simulink model "scdmechconveyor"  (Simulink 7.6)
settings: Solver=ode45  StartTime=0  StopTime=20  FixedStep=0.1  RelTol=1e-4  AbsTol=1e-6
model workspace (MAT data in the model file):
  Dk = [0 0 -1]
  Ck = [-0.0984238285661 -0.00713806743411 0.066683215581 0.191712430065 -0.740222532454]
  Bk = [-1142.96829869  0  0; -16827.8569202  22530.9100751  0; -891.017707814  1697.05627485  0; -295.52924747  169.705627485  0; -37.2617766448  6.32455532034  0]
  Ak = [-108.803869467  1  0  0  0; -1589.64026344  0  -597.440973765  -5974.40973765  17812.2483984; -84.8196529029  0  -50  -450  1341.6407865; -28.1326487378  0  0  -50  134.16407865; -3.54710230093  0  0  0  0]
  Dw = 800
  Cw = [-21.2132034356 -212.132034356 632.455532034]
  Bw = [1697.05627485; 169.705627485; 6.32455532034]
  Aw = [-50  -450  1341.6407865; 0  -50  134.16407865; 0  0  0]
  Dwinv = 0.00125
  Cwinv = [-0.0265165042945 -0.265165042945 0.790569415042]
  Bwinv = [-2.12132034356; -0.212132034356; -0.00790569415042]
  Awinv = [-5  0  0; 4.5  -5  0; 0.167705098312  1.67705098312  -5]
  Sig : Simulink.Signal (value not decoded)
values from neighbouring files (symbols this model uses):
  m = 0.1    [magballdat.m]
libraries: mblibv1 x18
settings Model: Creator=The MathWorks Inc.  ExtModeAutoUpdateStatusClock=off
settings SolverCC: InsertRTBMode=Auto
settings DataIOCC: SaveOutput=off  SaveTime=off  SignalLoggingName=scd_datalog
settings OptimizationCC: BooleanDataType=off  InlineInvariantSignals=on  InitFltsAndDblsToZero=on
settings DebuggingCC: AlgebraicLoopMsg=none  SaveWithParameterizedLinksMsg=none  CheckExecutionContextPreStartOutputMsg=on  CheckExecutionContextRuntimeOutputMsg=on  SignalResolutionControl=TryResolveAllWithWarning  SolverPrmCheckMsg=none  MultiTaskDSMMsg=warning  UnconnectedInputMsg=none  UnconnectedOutputMsg=none  UnconnectedLineMsg=none  InitInArrayFormatMsg=none  StrictBusMsg=None
settings HardwareCC: TargetUnknown=on
settings GRTTargetCC: TargetFcnLib=ansi_tfl_tmw.mat
settings SimMechanicsCC: WarnOnRedundantConstraints=off

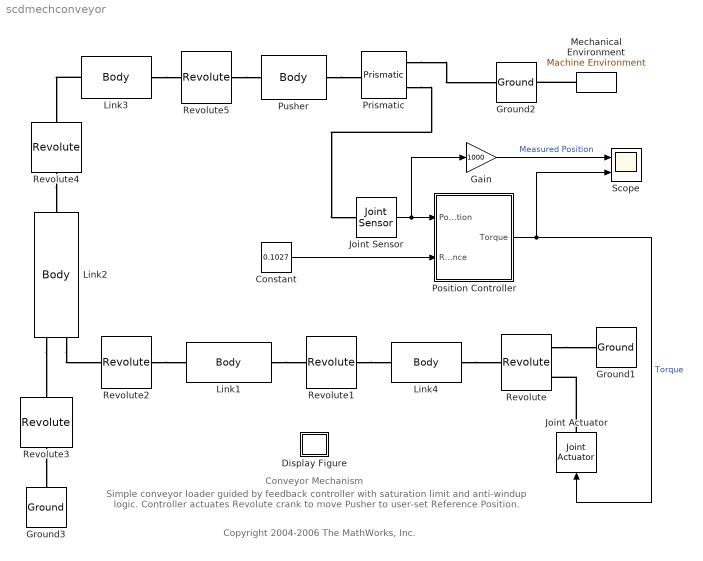
== system scdmechconveyor ==
  note: Conveyor Mechanism
  note: Simple conveyor loader guided by feedback controller with saturation limit
      | and anti-windup logic. Controller actuates Revolute crank to move Pusher
      | to user-set Reference Position.
  note: Copyright 2004-2006 The MathWorks, Inc.
  Constant : Constant  Value=0.1027
  Display Figure : Subsystem  Tag=Help  Description="Help callback for conveyor model: mech_conveyor.  Opens Help browser to Type 19 marker at documentation for this tutorial model."
      settings: OpenFcn=pmhelpview([docroot '/toolbox/physmod/mech/mech.map'], 'mech_conveyor_help');
      mask Type: Help callback
      mask Display: image(imread('info.bmp'))
  Gain : Gain  Gain=1000  SaturateOnIntegerOverflow=on  OutDataTypeStr=Inherit: Same as input  ParamDataTypeStr=Inherit: Same as input
  Ground1 : mblibv1/Bodies/Ground  DialogController=MECH.DynMechDlgSource  SystemSampleTime=-1  UpdateFromCAD=off  LeftPortType=env  RightPortType=workingframe  PhysicalDomain=Mechanical  DialogClass=GroundBlock  CoordPosition=[0.280 0.210 0]  CoordPositionUnits=m  StateVectorMgrId=-1  MachineId=[0 0]  ShowEnvPort=off
  Ground2 : mblibv1/Bodies/Ground  DialogController=MECH.DynMechDlgSource  SystemSampleTime=-1  UpdateFromCAD=off  LeftPortType=env  RightPortType=workingframe  PhysicalDomain=Mechanical  DialogClass=GroundBlock  CoordPosition=[0.412 0.5 0]  CoordPositionUnits=m  StateVectorMgrId=-1  MachineId=[0 0]  ShowEnvPort=on
  Ground3 : mblibv1/Bodies/Ground  DialogController=MECH.DynMechDlgSource  SystemSampleTime=-1  UpdateFromCAD=off  LeftPortType=env  RightPortType=workingframe  PhysicalDomain=Mechanical  DialogClass=GroundBlock  CoordPosition=[0.08 0.11 0]  CoordPositionUnits=m  StateVectorMgrId=-1  MachineId=[0 0]  ShowEnvPort=off
  Joint Actuator : mblibv1/Sensors &  Actuators/Joint Actuator  DialogController=MECH.DynMechDlgSource  SystemSampleTime=-1  UpdateFromCAD=off  PhysicalDomain=Mechanical  PortType=blob  ActuationStyle=Force  AngleUnits=rad  ArcVelocityUnits=rad/s  ArcAccelerationUnits=rad/s^2  CoordPositionUnits=m  VelocityUnits=m/s  AccelerationUnits=m/s^2  ForceUnits=N  TorqueUnits=N-m  ActiveIO=on  Width=1  DialogClass=MechanicalActuatorBlock  Primitive=R1  ReferenceFrame=Absolute (INERTIAL)
  Joint Sensor : mblibv1/Sensors &  Actuators/Joint Sensor  DialogController=MECH.DynMechDlgSource  SystemSampleTime=-1  UpdateFromCAD=off  PhysicalDomain=Mechanical  PortType=blob  Muxed=on  Pose=off  Angle=on  AngleUnits=deg  ArcVelocity=off  ArcVelocityUnits=deg/s  ArcAcceleration=off  ArcAccelerationUnits=deg/s^2  CoordPosition=on  CoordPositionUnits=m  Velocity=off  VelocityUnits=m/s  Acceleration=off  AccelerationUnits=m/s^2  Quaternion=on  QuaternionDT=off  QuaternionDDT=off  QuaternionUnits=off  OutputVector=[ 1 ]  ActiveIO=on  Width=1  DialogClass=MechanicalSensorBlock  Primitive=P1  Force=off  ForceUnits=N  Torque=off  TorqueUnits=N-m  ReferenceFrame=Absolute (INERTIAL)  ReactionSensedSide=Base  ReactionReferenceFrame=Absolute (World)  ReactionForce=off  ReactionForceUnits=N  ReactionMoment=off  ReactionMomentUnits=N-m
  Link1 : mblibv1/Bodies/Body  DialogController=MECH.DynMechDlgSource  PhysicalDomain=mechanical  SubClassName=Unknown  LeftPortType=workingframe  RightPortType=workingframe  LConnTagsString=CS1  RConnTagsString=CS2  UpdateFromCAD=off  DialogClass=MechanicalBodyBlock  Mass=0.98785  MassUnits=kg  InertiaUnits=kg*m^2  Inertia=[7.6414e-005 -9.2222e-005 1.8971e-009;-9.2222e-005 0.0083286 -2.5235e-010;1.8971e-009 -2.5235e-010 0.0083397]  Shape=Cylinder  ShapeDims=[1 1]  ShapeUnits=m  ShapeUse=false  Density=1  DensityUnits=kg/m^3  DensityUse=false  GraphicsMode=1  BodyColorSelMode=MACHINE_DEFAULT  BodyColor=[0.5 0.5 0.5]  AttachedToCS=1  CG=Left$CG$[0.110 0.247 0]$WORLD$WORLD$m$[0 0 -4.22]$Euler X-Y-Z$deg$WORLD$false  WorkingFrames=Left$CS1$[0.265 0.236 0]$WORLD$WORLD$m$[0 0 0]$Euler X-Y-Z$deg$WORLD$true#Right$CS2$[-0.299 0.022 0]$WORLD$CS1$m$[0 0 0]$Euler X-Y-Z$deg$WORLD$true  CGPos=[0.110 0.247 0]  CGRot=[0 0 -4.22]  CS0Pos=[]  CS0Rot=[]  CS1Pos=[0.265 0.236 0]  CS1Rot=[0 0 0]  CS2Pos=[-0.299 0.022 0]  CS2Rot=[0 0 0]  CS3Pos=[]  CS3Rot=[]  CS4Pos=[]  CS4Rot=[]  CS5Pos=[]  CS5Rot=[]  CS6Pos=[]  CS6Rot=[]  CS7Pos=[]  CS7Rot=[]  CS8Pos=[]  CS8Rot=[]  CS9Pos=[]  CS9Rot=[]  CS10Pos=[]  CS10Rot=[]  CS11Pos=[]  CS11Rot=[]  CS12Pos=[]  CS12Rot=[]  CS13Pos=[]  CS13Rot=[]  CS14Pos=[]  CS14Rot=[]  CS15Pos=[]  CS15Rot=[]  CS16Pos=[]  CS16Rot=[]  CS17Pos=[]  CS17Rot=[]  CS18Pos=[]  CS18Rot=[]  CS19Pos=[]  CS19Rot=[]  CS20Pos=[]  CS20Rot=[]
  Link2 : mblibv1/Bodies/Body  DialogController=MECH.DynMechDlgSource  PhysicalDomain=mechanical  SubClassName=Unknown  LeftPortType=workingframe  RightPortType=workingframe  LConnTagsString=CS1|CS2  RConnTagsString=CS3  UpdateFromCAD=off  DialogClass=MechanicalBodyBlock  Mass=2.7433  MassUnits=kg  InertiaUnits=kg*m^2  Inertia=[0.0044915 2.9472e-005 1.0996e-007;2.9472e-005 0.089001 -4.3534e-007;1.0996e-007 -4.3534e-007 0.093312]  Shape=Cylinder  ShapeDims=[1 1]  ShapeUnits=m  ShapeUse=false  Density=1  DensityUnits=kg/m^3  DensityUse=false  GraphicsMode=1  BodyColorSelMode=MACHINE_DEFAULT  BodyColor=[0.5 0.5 0.5]  AttachedToCS=1  CG=Left$CG$[-0.030 0.402 0]$WORLD$WORLD$m$[0 0 95.31]$Euler X-Y-Z$deg$WORLD$false  WorkingFrames=Left$CS1$[0.08 0.11 0]$WORLD$WORLD$m$[0 0 0]$Euler X-Y-Z$deg$WORLD$true#Left$CS2$[-0.114 0.148 0]$WORLD$CS1$m$[0 0 0]$Euler X-Y-Z$deg$WORLD$true#Right$CS3$[0.059 0.449 0]$WORLD$CS2$m$[0 0 0]$Euler X-Y-Z$deg$WORLD$true  CGPos=[-0.030 0.402 0]  CGRot=[0 0 95.31]  CS0Pos=[]  CS0Rot=[]  CS1Pos=[0.08 0.11 0]  CS1Rot=[0 0 0]  CS2Pos=[-0.114 0.148 0]  CS2Rot=[0 0 0]  CS3Pos=[0.059 0.449 0]  CS3Rot=[0 0 0]  CS4Pos=[]  CS4Rot=[]  CS5Pos=[]  CS5Rot=[]  CS6Pos=[]  CS6Rot=[]  CS7Pos=[]  CS7Rot=[]  CS8Pos=[]  CS8Rot=[]  CS9Pos=[]  CS9Rot=[]  CS10Pos=[]  CS10Rot=[]  CS11Pos=[]  CS11Rot=[]  CS12Pos=[]  CS12Rot=[]  CS13Pos=[]  CS13Rot=[]  CS14Pos=[]  CS14Rot=[]  CS15Pos=[]  CS15Rot=[]  CS16Pos=[]  CS16Rot=[]  CS17Pos=[]  CS17Rot=[]  CS18Pos=[]  CS18Rot=[]  CS19Pos=[]  CS19Rot=[]  CS20Pos=[]  CS20Rot=[]
  Link3 : mblibv1/Bodies/Body  DialogController=MECH.DynMechDlgSource  PhysicalDomain=mechanical  SubClassName=Unknown  LeftPortType=workingframe  RightPortType=workingframe  LConnTagsString=CS1  RConnTagsString=CS2  UpdateFromCAD=off  DialogClass=MechanicalBodyBlock  Mass=1.2355  MassUnits=kg  InertiaUnits=kg*m^2  Inertia=[8.2129e-005 1.8216e-005 -3.7069e-010;1.8216e-005 0.017391 -2.6914e-011;-3.7069e-010 -2.6914e-011 0.017392]  Shape=Cylinder  ShapeDims=[1 1]  ShapeUnits=m  ShapeUse=false  Density=1  DensityUnits=kg/m^3  DensityUse=false  GraphicsMode=1  BodyColorSelMode=MACHINE_DEFAULT  BodyColor=[0.5 0.5 0.5]  AttachedToCS=1  CG=Left$CG$[0.194 0.604 0.01]$WORLD$WORLD$m$[90 -31.24 0]$Euler X-Y-Z$deg$WORLD$false  WorkingFrames=Left$CS1$[0.025 0.707 0]$WORLD$WORLD$m$[0 0 0]$Euler X-Y-Z$deg$WORLD$true#Right$CS2$[0.342 -0.207 0]$WORLD$CS1$m$[0 0 0]$Euler X-Y-Z$deg$WORLD$true  CGPos=[0.194 0.604 0.01]  CGRot=[90 -31.24 0]  CS0Pos=[]  CS0Rot=[]  CS1Pos=[0.025 0.707 0]  CS1Rot=[0 0 0]  CS2Pos=[0.342 -0.207 0]  CS2Rot=[0 0 0]  CS3Pos=[]  CS3Rot=[]  CS4Pos=[]  CS4Rot=[]  CS5Pos=[]  CS5Rot=[]  CS6Pos=[]  CS6Rot=[]  CS7Pos=[]  CS7Rot=[]  CS8Pos=[]  CS8Rot=[]  CS9Pos=[]  CS9Rot=[]  CS10Pos=[]  CS10Rot=[]  CS11Pos=[]  CS11Rot=[]  CS12Pos=[]  CS12Rot=[]  CS13Pos=[]  CS13Rot=[]  CS14Pos=[]  CS14Rot=[]  CS15Pos=[]  CS15Rot=[]  CS16Pos=[]  CS16Rot=[]  CS17Pos=[]  CS17Rot=[]  CS18Pos=[]  CS18Rot=[]  CS19Pos=[]  CS19Rot=[]  CS20Pos=[]  CS20Rot=[]
  Link4 : mblibv1/Bodies/Body  DialogController=MECH.DynMechDlgSource  PhysicalDomain=mechanical  SubClassName=Unknown  LeftPortType=workingframe  RightPortType=workingframe  LConnTagsString=CS1  RConnTagsString=CS2  UpdateFromCAD=off  DialogClass=MechanicalBodyBlock  Mass=0.057538  MassUnits=kg  InertiaUnits=kg*m^2  Inertia=[1.0148e-005 0 0;0 2.5218e-006 0;0 0 1.1711e-005]  Shape=Cylinder  ShapeDims=[1 1]  ShapeUnits=m  ShapeUse=false  Density=1  DensityUnits=kg/m^3  DensityUse=false  GraphicsMode=1  BodyColorSelMode=MACHINE_DEFAULT  BodyColor=[0.5 0.5 0.5]  AttachedToCS=1  CG=Left$CG$[0.272 0.223 0.01]$WORLD$WORLD$m$[0 0 30]$Euler X-Y-Z$deg$WORLD$false  WorkingFrames=Left$CS1$[0.280 0.210 0]$WORLD$WORLD$m$[0 0 0]$Euler X-Y-Z$deg$WORLD$true#Right$CS2$[-0.015 0.026 0]$CS1$CS1$m$[0 0 0]$Euler X-Y-Z$deg$WORLD$true  CGPos=[0.272 0.223 0.01]  CGRot=[0 0 30]  CS0Pos=[]  CS0Rot=[]  CS1Pos=[0.280 0.210 0]  CS1Rot=[0 0 0]  CS2Pos=[-0.015 0.026 0]  CS2Rot=[0 0 0]  CS3Pos=[]  CS3Rot=[]  CS4Pos=[]  CS4Rot=[]  CS5Pos=[]  CS5Rot=[]  CS6Pos=[]  CS6Rot=[]  CS7Pos=[]  CS7Rot=[]  CS8Pos=[]  CS8Rot=[]  CS9Pos=[]  CS9Rot=[]  CS10Pos=[]  CS10Rot=[]  CS11Pos=[]  CS11Rot=[]  CS12Pos=[]  CS12Rot=[]  CS13Pos=[]  CS13Rot=[]  CS14Pos=[]  CS14Rot=[]  CS15Pos=[]  CS15Rot=[]  CS16Pos=[]  CS16Rot=[]  CS17Pos=[]  CS17Rot=[]  CS18Pos=[]  CS18Rot=[]  CS19Pos=[]  CS19Rot=[]  CS20Pos=[]  CS20Rot=[]
  Mechanical Environment : mblibv1/Bodies/Machine Environment  Tag=Factory ground  DialogController=MECH.DialogSource  SystemSampleTime=-1  PortType=env  PhysicalDomain=Mechanical  DialogTemplateClass=MECH.MachineEnvironment  SyncWhenCopied=off  Gravity=[0 -9.81 0]  GravityUnits=m/s^2  GravityAsSignal=off  Dimensionality=3D Only  AnalysisType=Forward dynamics  LinearAssemblyTolerance=1e-3  LinearAssemblyToleranceUnits=m  AngularAssemblyTolerance=1e-3  AngularAssemblyToleranceUnits=rad  ConstraintSolverType=Stabilizing  ConstraintRelTolerance=1e-4  ConstraintAbsTolerance=1e-4  UseRobustSingularityHandling=off  RedundancyAnalysisToleranceType=Automatically select tolerance  RedundancyAnalysisTolerance=1e-14  StatePerturbationType=Adaptive  PerturbationSize=1e-3  VisualizeMachine=off  BodyVisualizationType=Use model default body geometries  BodyColorSelMode=Use model default  DefaultBodyColor=[1 0 0]
  Position Controller : Subsystem
  Prismatic : mblibv1/Joints/Prismatic  DialogController=MECH.DynMechDlgSource  PhysicalDomain=mechanical  SubClassName=Unknown  LeftPortType=blob  RightPortType=blob  LConnTagsString=__newl0|SA1  RConnTagsString=__newr0  UpdateFromCAD=off  NumSAPorts=1  CutJoint=off  MarkAsCut=off  Primitives=prismatic  PrimitiveProps=P1$WORLD$[1 0 0]$prismatic  DialogClass=JointBlock  P1Axis=[1 0 0]
  Pusher : mblibv1/Bodies/Body  DialogController=MECH.DynMechDlgSource  PhysicalDomain=mechanical  SubClassName=Unknown  LeftPortType=workingframe  RightPortType=workingframe  LConnTagsString=CS1  RConnTagsString=CS2  UpdateFromCAD=off  DialogClass=MechanicalBodyBlock  Mass=1.8547  MassUnits=kg  InertiaUnits=kg*m^2  Inertia=[0.0025031 -1.671e-006 5.5014e-006;-1.671e-006 0.0016406 -1.8596e-007;5.5014e-006 -1.8596e-007 0.0011862]  Shape=Cylinder  ShapeDims=[1 1]  ShapeUnits=m  ShapeUse=false  Density=1  DensityUnits=kg/m^3  DensityUse=false  GraphicsMode=1  BodyColorSelMode=MACHINE_DEFAULT  BodyColor=[0.5 0.5 0.5]  AttachedToCS=1  CG=Left$CG$[0.396 0.499 0]$WORLD$WORLD$m$[0 0 0]$Euler X-Y-Z$deg$WORLD$false  WorkingFrames=Left$CS1$[0.367 0.5 0]$WORLD$WORLD$m$[0 0 0]$Euler X-Y-Z$deg$WORLD$true#Right$CS2$[0.045 0 0]$WORLD$CS1$m$[0 0 0]$Euler X-Y-Z$deg$WORLD$true  CGPos=[0.396 0.499 0]  CGRot=[0 0 0]  CS0Pos=[]  CS0Rot=[]  CS1Pos=[0.367 0.5 0]  CS1Rot=[0 0 0]  CS2Pos=[0.045 0 0]  CS2Rot=[0 0 0]  CS3Pos=[]  CS3Rot=[]  CS4Pos=[]  CS4Rot=[]  CS5Pos=[]  CS5Rot=[]  CS6Pos=[]  CS6Rot=[]  CS7Pos=[]  CS7Rot=[]  CS8Pos=[]  CS8Rot=[]  CS9Pos=[]  CS9Rot=[]  CS10Pos=[]  CS10Rot=[]  CS11Pos=[]  CS11Rot=[]  CS12Pos=[]  CS12Rot=[]  CS13Pos=[]  CS13Rot=[]  CS14Pos=[]  CS14Rot=[]  CS15Pos=[]  CS15Rot=[]  CS16Pos=[]  CS16Rot=[]  CS17Pos=[]  CS17Rot=[]  CS18Pos=[]  CS18Rot=[]  CS19Pos=[]  CS19Rot=[]  CS20Pos=[]  CS20Rot=[]
  Revolute : mblibv1/Joints/Revolute  DialogController=MECH.DynMechDlgSource  PhysicalDomain=mechanical  SubClassName=Unknown  LeftPortType=blob  RightPortType=blob  LConnTagsString=__newl0|SA1  RConnTagsString=__newr0  UpdateFromCAD=off  NumSAPorts=1  CutJoint=off  MarkAsCut=off  Primitives=revolute  PrimitiveProps=R1$WORLD$[0 0 1]$revolute  DialogClass=JointBlock  R1Axis=[0 0 1]
  Revolute1 : mblibv1/Joints/Revolute  DialogController=MECH.DynMechDlgSource  PhysicalDomain=mechanical  SubClassName=Unknown  LeftPortType=blob  RightPortType=blob  LConnTagsString=__newl0  RConnTagsString=__newr0  UpdateFromCAD=off  NumSAPorts=0  CutJoint=off  MarkAsCut=off  Primitives=revolute  PrimitiveProps=R1$WORLD$[0 0 1]$revolute  DialogClass=JointBlock  R1Axis=[0 0 1]
  Revolute2 : mblibv1/Joints/Revolute  DialogController=MECH.DynMechDlgSource  PhysicalDomain=mechanical  SubClassName=Unknown  LeftPortType=blob  RightPortType=blob  LConnTagsString=__newl0  RConnTagsString=__newr0  UpdateFromCAD=off  NumSAPorts=0  CutJoint=on  MarkAsCut=off  Primitives=revolute  PrimitiveProps=R1$WORLD$[0 0 1]$revolute  DialogClass=JointBlock  R1Axis=[0 0 1]
  Revolute3 : mblibv1/Joints/Revolute  DialogController=MECH.DynMechDlgSource  PhysicalDomain=mechanical  SubClassName=Unknown  LeftPortType=blob  RightPortType=blob  LConnTagsString=__newl0  RConnTagsString=__newr0  UpdateFromCAD=off  NumSAPorts=0  CutJoint=off  MarkAsCut=off  Primitives=revolute  PrimitiveProps=R1$WORLD$[0 0 1]$revolute  DialogClass=JointBlock  R1Axis=[0 0 1]
  Revolute4 : mblibv1/Joints/Revolute  DialogController=MECH.DynMechDlgSource  PhysicalDomain=mechanical  SubClassName=Unknown  LeftPortType=blob  RightPortType=blob  LConnTagsString=__newl0  RConnTagsString=__newr0  UpdateFromCAD=off  NumSAPorts=0  CutJoint=on  MarkAsCut=off  Primitives=revolute  PrimitiveProps=R1$WORLD$[0 0 1]$revolute  DialogClass=JointBlock  R1Axis=[0 0 1]
  Revolute5 : mblibv1/Joints/Revolute  DialogController=MECH.DynMechDlgSource  PhysicalDomain=mechanical  SubClassName=Unknown  LeftPortType=blob  RightPortType=blob  LConnTagsString=__newl0  RConnTagsString=__newr0  UpdateFromCAD=off  NumSAPorts=0  CutJoint=off  MarkAsCut=off  Primitives=revolute  PrimitiveProps=R1$WORLD$[0 0 1]$revolute  DialogClass=JointBlock  R1Axis=[0 0 1]
  Scope : Scope  NumInputPorts=2
      settings: TimeRange=20  YMin=0~-5  YMax=110~0.5
  wires:
  Joint Sensor/1 -> Position Controller/1(Position), Gain/1
  Constant/1 -> Position Controller/2(Reference)
  Position Controller/1(Torque) -> Joint Actuator/1, Scope/2  "Torque"
  Gain/1 -> Scope/1  "Measured Position"
  connections:
  Link2/LConn1 -- Revolute3/RConn1
  Revolute3/LConn1 -- Ground3/RConn1
  Revolute4/LConn1 -- Link2/RConn1
  Link2/LConn2 -- Revolute2/RConn1
  Link3/LConn1 -- Revolute4/RConn1
  Link3/RConn1 -- Revolute5/LConn1
  Revolute5/RConn1 -- Pusher/LConn1
  Revolute2/LConn1 -- Link1/RConn1
  Link1/LConn1 -- Revolute1/RConn1
  Revolute1/LConn1 -- Link4/RConn1
  Link4/LConn1 -- Revolute/RConn1
  Revolute/LConn1 -- Ground1/RConn1
  Prismatic/LConn2 -- Joint Sensor/LConn1
  Joint Actuator/RConn1 -- Revolute/LConn2
  Prismatic/LConn1 -- Ground2/RConn1
  Pusher/RConn1 -- Prismatic/RConn1
  Mechanical Environment/RConn1 -- Ground2/LConn1

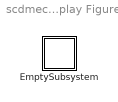
== system scdmechconveyor/Display Figure ==
  EmptySubsystem : Subsystem

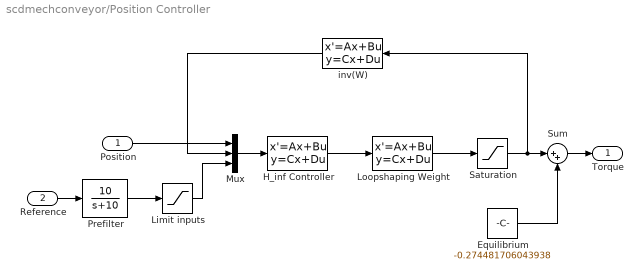
== system scdmechconveyor/Position Controller ==
  Position : Inport
  Reference : Inport  Port=2
  Equilibrium : Constant  Value=-0.274481706043938
  H_inf Controller : StateSpace  A=Ak  B=Bk  C=Ck  D=Dk
  Limit inputs : Saturate  UpperLimit=0.2  LowerLimit=0
  Loopshaping Weight : StateSpace  A=Aw  B=Bw  C=Cw  D=Dw
  Mux : Mux  Inputs=3
  Prefilter : TransferFcn  Numerator=[10]  Denominator=[1 10]
  Saturation : Saturate  UpperLimit=5  LowerLimit=-5+0.7647
  Sum : Sum  Inputs=|++  SaturateOnIntegerOverflow=on  InputSameDT=on  OutDataTypeStr=Inherit: Same as first input
  inv(W) : StateSpace  A=Awinv  B=Bwinv  C=Cwinv  D=Dwinv
  Torque : Outport
  wires:
  H_inf Controller/1 -> Loopshaping Weight/1
  Mux/1 -> H_inf Controller/1
  Position/1 -> Mux/1
  Limit inputs/1 -> Mux/3
  inv(W)/1 -> Mux/2
  Loopshaping Weight/1 -> Saturation/1
  Saturation/1 -> Sum/1, inv(W)/1
  Sum/1 -> Torque/1
  Equilibrium/1 -> Sum/2
  Prefilter/1 -> Limit inputs/1
  Reference/1 -> Prefilter/1

== system scdmechconveyor/Display Figure/EmptySubsystem ==
